simulink model "stewart_platform"  (R2013a)
settings: Solver=ode45  StartTime=0.0  StopTime=10.0  RelTol=1e-3
undefined symbols (not defined in the file): X, Y, Z
libraries: sm_lib x1374, nesl_utility x1
(part 22 of 30)

== system stewart_platform/ActuatorAssm4_2/DrivenAssm_1_RIGID/Recessed_Pan_Head_Screw_M2x8_48_Z_3_RIGID ==
  ReferenceFrame : sm_lib/Frames and  Transforms/Reference  Frame  BlockFunction=simmechanics.library.frames_transforms.reference_frame
  Solid : sm_lib/Body Elements/Solid  InertiaType=Custom  Mass=0.00030420099999999998  MassUnits=kg  CenterOfMass=[0.23057999999999998 -4.2158300000000003e-10 -1.6472500000000001e-11]  CenterOfMassUnits=cm  MomentsOfInertia=[3.0540999999999997e-06 2.6916499999999999e-05 2.6916499999999999e-05]  MomentsOfInertiaUnits=kg*cm^2  ProductsOfInertia=[0 0 0]  ProductsOfInertiaUnits=kg*cm^2  DensityBased=on  Density=1000  DensityUnits=kg/(m^3)  GraphicType=FromGeometry  MarkerShape=Sphere  MarkerSize=10  MarkerSizeUnits=m  GraphicVisPropType=SimpleVisualProperties  GraphicDiffuseColor=[0.722824 0.722824 0.722824]  GraphicSpecularColor=[0.5 0.5 0.5 1.0]  GraphicAmbientColor=[0.15 0.15 0.15 1.0]  GraphicEmissiveColor=[0.0 0.0 0.0 1.0]  GraphicShininess=75  GraphicOpacity=1  GeometryShape=FromFile  RectangleSize=[1 1]  RectangleSizeUnits=m  BrickDimensions=[1 1 1]  BrickDimensionUnits=m  CylinderRadius=1  CylinderRadiusUnits=m  CylinderLength=1  CylinderLengthUnits=m  SphereRadius=1  SphereRadiusUnits=m  EllipsoidRadii=[1 1 1]  EllipsoidRadiiUnits=m  ExtrusionCrossSection=[1 1; -1 1; -1 -1; 1 -1]  ExtrusionCrossSectionUnits=m  ExtrusionLength=1  ExtrusionLengthUnits=m  PolygonNumSides=3  PolygonOuterRadius=1  PolygonOuterRadiusUnits=m  ExtGeomFileName=Recessed_Pan_Head_Screw_M2x8_48_Z_Default_sldprt.STL  ExtGeomFileUnits=cm  RevolutionCrossSection=[1 1; 1 -1; 2 -1; 2 1]  RevolutionCrossSectionUnits=m  RevolutionExtent=Full  RevolutionAngle=180  RevolutionAngleUnits=deg  BlockFunction=simmechanics.library.body_elements.solid
  F : PMIOPort  Port=1  Side=Left
  connections:
  Solid/RConn1 -- ReferenceFrame/RConn1 -- F/RConn1

== system stewart_platform/ActuatorAssm4_2/DrivenAssm_1_RIGID/Recessed_Pan_Head_Screw_M2x8_48_Z_4_RIGID ==
  ReferenceFrame : sm_lib/Frames and  Transforms/Reference  Frame  BlockFunction=simmechanics.library.frames_transforms.reference_frame
  Solid : sm_lib/Body Elements/Solid  InertiaType=Custom  Mass=0.00030420099999999998  MassUnits=kg  CenterOfMass=[0.23057999999999998 -4.2158300000000003e-10 -1.6472500000000001e-11]  CenterOfMassUnits=cm  MomentsOfInertia=[3.0540999999999997e-06 2.6916499999999999e-05 2.6916499999999999e-05]  MomentsOfInertiaUnits=kg*cm^2  ProductsOfInertia=[0 0 0]  ProductsOfInertiaUnits=kg*cm^2  DensityBased=on  Density=1000  DensityUnits=kg/(m^3)  GraphicType=FromGeometry  MarkerShape=Sphere  MarkerSize=10  MarkerSizeUnits=m  GraphicVisPropType=SimpleVisualProperties  GraphicDiffuseColor=[0.722824 0.722824 0.722824]  GraphicSpecularColor=[0.5 0.5 0.5 1.0]  GraphicAmbientColor=[0.15 0.15 0.15 1.0]  GraphicEmissiveColor=[0.0 0.0 0.0 1.0]  GraphicShininess=75  GraphicOpacity=1  GeometryShape=FromFile  RectangleSize=[1 1]  RectangleSizeUnits=m  BrickDimensions=[1 1 1]  BrickDimensionUnits=m  CylinderRadius=1  CylinderRadiusUnits=m  CylinderLength=1  CylinderLengthUnits=m  SphereRadius=1  SphereRadiusUnits=m  EllipsoidRadii=[1 1 1]  EllipsoidRadiiUnits=m  ExtrusionCrossSection=[1 1; -1 1; -1 -1; 1 -1]  ExtrusionCrossSectionUnits=m  ExtrusionLength=1  ExtrusionLengthUnits=m  PolygonNumSides=3  PolygonOuterRadius=1  PolygonOuterRadiusUnits=m  ExtGeomFileName=Recessed_Pan_Head_Screw_M2x8_48_Z_Default_sldprt.STL  ExtGeomFileUnits=cm  RevolutionCrossSection=[1 1; 1 -1; 2 -1; 2 1]  RevolutionCrossSectionUnits=m  RevolutionExtent=Full  RevolutionAngle=180  RevolutionAngleUnits=deg  BlockFunction=simmechanics.library.body_elements.solid
  F : PMIOPort  Port=1  Side=Left
  connections:
  Solid/RConn1 -- ReferenceFrame/RConn1 -- F/RConn1

== system stewart_platform/ActuatorAssm4_2/DrivenAssm_1_RIGID/Recessed_Pan_Head_Screw_M2x8_48_Z_5_RIGID ==
  ReferenceFrame : sm_lib/Frames and  Transforms/Reference  Frame  BlockFunction=simmechanics.library.frames_transforms.reference_frame
  Solid : sm_lib/Body Elements/Solid  InertiaType=Custom  Mass=0.00030420099999999998  MassUnits=kg  CenterOfMass=[0.23057999999999998 -4.2158300000000003e-10 -1.6472500000000001e-11]  CenterOfMassUnits=cm  MomentsOfInertia=[3.0540999999999997e-06 2.6916499999999999e-05 2.6916499999999999e-05]  MomentsOfInertiaUnits=kg*cm^2  ProductsOfInertia=[0 0 0]  ProductsOfInertiaUnits=kg*cm^2  DensityBased=on  Density=1000  DensityUnits=kg/(m^3)  GraphicType=FromGeometry  MarkerShape=Sphere  MarkerSize=10  MarkerSizeUnits=m  GraphicVisPropType=SimpleVisualProperties  GraphicDiffuseColor=[0.722824 0.722824 0.722824]  GraphicSpecularColor=[0.5 0.5 0.5 1.0]  GraphicAmbientColor=[0.15 0.15 0.15 1.0]  GraphicEmissiveColor=[0.0 0.0 0.0 1.0]  GraphicShininess=75  GraphicOpacity=1  GeometryShape=FromFile  RectangleSize=[1 1]  RectangleSizeUnits=m  BrickDimensions=[1 1 1]  BrickDimensionUnits=m  CylinderRadius=1  CylinderRadiusUnits=m  CylinderLength=1  CylinderLengthUnits=m  SphereRadius=1  SphereRadiusUnits=m  EllipsoidRadii=[1 1 1]  EllipsoidRadiiUnits=m  ExtrusionCrossSection=[1 1; -1 1; -1 -1; 1 -1]  ExtrusionCrossSectionUnits=m  ExtrusionLength=1  ExtrusionLengthUnits=m  PolygonNumSides=3  PolygonOuterRadius=1  PolygonOuterRadiusUnits=m  ExtGeomFileName=Recessed_Pan_Head_Screw_M2x8_48_Z_Default_sldprt.STL  ExtGeomFileUnits=cm  RevolutionCrossSection=[1 1; 1 -1; 2 -1; 2 1]  RevolutionCrossSectionUnits=m  RevolutionExtent=Full  RevolutionAngle=180  RevolutionAngleUnits=deg  BlockFunction=simmechanics.library.body_elements.solid
  F : PMIOPort  Port=1  Side=Left
  connections:
  Solid/RConn1 -- ReferenceFrame/RConn1 -- F/RConn1

== system stewart_platform/ActuatorAssm4_2/DrivenAssm_1_RIGID/Recessed_Pan_Head_Screw_M2x8_48_Z_6_RIGID ==
  ReferenceFrame : sm_lib/Frames and  Transforms/Reference  Frame  BlockFunction=simmechanics.library.frames_transforms.reference_frame
  Solid : sm_lib/Body Elements/Solid  InertiaType=Custom  Mass=0.00030420099999999998  MassUnits=kg  CenterOfMass=[0.23057999999999998 -4.2158300000000003e-10 -1.6472500000000001e-11]  CenterOfMassUnits=cm  MomentsOfInertia=[3.0540999999999997e-06 2.6916499999999999e-05 2.6916499999999999e-05]  MomentsOfInertiaUnits=kg*cm^2  ProductsOfInertia=[0 0 0]  ProductsOfInertiaUnits=kg*cm^2  DensityBased=on  Density=1000  DensityUnits=kg/(m^3)  GraphicType=FromGeometry  MarkerShape=Sphere  MarkerSize=10  MarkerSizeUnits=m  GraphicVisPropType=SimpleVisualProperties  GraphicDiffuseColor=[0.722824 0.722824 0.722824]  GraphicSpecularColor=[0.5 0.5 0.5 1.0]  GraphicAmbientColor=[0.15 0.15 0.15 1.0]  GraphicEmissiveColor=[0.0 0.0 0.0 1.0]  GraphicShininess=75  GraphicOpacity=1  GeometryShape=FromFile  RectangleSize=[1 1]  RectangleSizeUnits=m  BrickDimensions=[1 1 1]  BrickDimensionUnits=m  CylinderRadius=1  CylinderRadiusUnits=m  CylinderLength=1  CylinderLengthUnits=m  SphereRadius=1  SphereRadiusUnits=m  EllipsoidRadii=[1 1 1]  EllipsoidRadiiUnits=m  ExtrusionCrossSection=[1 1; -1 1; -1 -1; 1 -1]  ExtrusionCrossSectionUnits=m  ExtrusionLength=1  ExtrusionLengthUnits=m  PolygonNumSides=3  PolygonOuterRadius=1  PolygonOuterRadiusUnits=m  ExtGeomFileName=Recessed_Pan_Head_Screw_M2x8_48_Z_Default_sldprt.STL  ExtGeomFileUnits=cm  RevolutionCrossSection=[1 1; 1 -1; 2 -1; 2 1]  RevolutionCrossSectionUnits=m  RevolutionExtent=Full  RevolutionAngle=180  RevolutionAngleUnits=deg  BlockFunction=simmechanics.library.body_elements.solid
  F : PMIOPort  Port=1  Side=Left
  connections:
  Solid/RConn1 -- ReferenceFrame/RConn1 -- F/RConn1

== system stewart_platform/ActuatorAssm4_2/DrivenAssm_1_RIGID/Recessed_Pan_Head_Screw_M2x8_48_Z_7_RIGID ==
  ReferenceFrame : sm_lib/Frames and  Transforms/Reference  Frame  BlockFunction=simmechanics.library.frames_transforms.reference_frame
  Solid : sm_lib/Body Elements/Solid  InertiaType=Custom  Mass=0.00030420099999999998  MassUnits=kg  CenterOfMass=[0.23057999999999998 -4.2158300000000003e-10 -1.6472500000000001e-11]  CenterOfMassUnits=cm  MomentsOfInertia=[3.0540999999999997e-06 2.6916499999999999e-05 2.6916499999999999e-05]  MomentsOfInertiaUnits=kg*cm^2  ProductsOfInertia=[0 0 0]  ProductsOfInertiaUnits=kg*cm^2  DensityBased=on  Density=1000  DensityUnits=kg/(m^3)  GraphicType=FromGeometry  MarkerShape=Sphere  MarkerSize=10  MarkerSizeUnits=m  GraphicVisPropType=SimpleVisualProperties  GraphicDiffuseColor=[0.722824 0.722824 0.722824]  GraphicSpecularColor=[0.5 0.5 0.5 1.0]  GraphicAmbientColor=[0.15 0.15 0.15 1.0]  GraphicEmissiveColor=[0.0 0.0 0.0 1.0]  GraphicShininess=75  GraphicOpacity=1  GeometryShape=FromFile  RectangleSize=[1 1]  RectangleSizeUnits=m  BrickDimensions=[1 1 1]  BrickDimensionUnits=m  CylinderRadius=1  CylinderRadiusUnits=m  CylinderLength=1  CylinderLengthUnits=m  SphereRadius=1  SphereRadiusUnits=m  EllipsoidRadii=[1 1 1]  EllipsoidRadiiUnits=m  ExtrusionCrossSection=[1 1; -1 1; -1 -1; 1 -1]  ExtrusionCrossSectionUnits=m  ExtrusionLength=1  ExtrusionLengthUnits=m  PolygonNumSides=3  PolygonOuterRadius=1  PolygonOuterRadiusUnits=m  ExtGeomFileName=Recessed_Pan_Head_Screw_M2x8_48_Z_Default_sldprt.STL  ExtGeomFileUnits=cm  RevolutionCrossSection=[1 1; 1 -1; 2 -1; 2 1]  RevolutionCrossSectionUnits=m  RevolutionExtent=Full  RevolutionAngle=180  RevolutionAngleUnits=deg  BlockFunction=simmechanics.library.body_elements.solid
  F : PMIOPort  Port=1  Side=Left
  connections:
  Solid/RConn1 -- ReferenceFrame/RConn1 -- F/RConn1

== system stewart_platform/ActuatorAssm4_2/DrivenAssm_1_RIGID/Recessed_Pan_Head_Screw_M2x8_48_Z_8_RIGID ==
  ReferenceFrame : sm_lib/Frames and  Transforms/Reference  Frame  BlockFunction=simmechanics.library.frames_transforms.reference_frame
  Solid : sm_lib/Body Elements/Solid  InertiaType=Custom  Mass=0.00030420099999999998  MassUnits=kg  CenterOfMass=[0.23057999999999998 -4.2158300000000003e-10 -1.6472500000000001e-11]  CenterOfMassUnits=cm  MomentsOfInertia=[3.0540999999999997e-06 2.6916499999999999e-05 2.6916499999999999e-05]  MomentsOfInertiaUnits=kg*cm^2  ProductsOfInertia=[0 0 0]  ProductsOfInertiaUnits=kg*cm^2  DensityBased=on  Density=1000  DensityUnits=kg/(m^3)  GraphicType=FromGeometry  MarkerShape=Sphere  MarkerSize=10  MarkerSizeUnits=m  GraphicVisPropType=SimpleVisualProperties  GraphicDiffuseColor=[0.722824 0.722824 0.722824]  GraphicSpecularColor=[0.5 0.5 0.5 1.0]  GraphicAmbientColor=[0.15 0.15 0.15 1.0]  GraphicEmissiveColor=[0.0 0.0 0.0 1.0]  GraphicShininess=75  GraphicOpacity=1  GeometryShape=FromFile  RectangleSize=[1 1]  RectangleSizeUnits=m  BrickDimensions=[1 1 1]  BrickDimensionUnits=m  CylinderRadius=1  CylinderRadiusUnits=m  CylinderLength=1  CylinderLengthUnits=m  SphereRadius=1  SphereRadiusUnits=m  EllipsoidRadii=[1 1 1]  EllipsoidRadiiUnits=m  ExtrusionCrossSection=[1 1; -1 1; -1 -1; 1 -1]  ExtrusionCrossSectionUnits=m  ExtrusionLength=1  ExtrusionLengthUnits=m  PolygonNumSides=3  PolygonOuterRadius=1  PolygonOuterRadiusUnits=m  ExtGeomFileName=Recessed_Pan_Head_Screw_M2x8_48_Z_Default_sldprt.STL  ExtGeomFileUnits=cm  RevolutionCrossSection=[1 1; 1 -1; 2 -1; 2 1]  RevolutionCrossSectionUnits=m  RevolutionExtent=Full  RevolutionAngle=180  RevolutionAngleUnits=deg  BlockFunction=simmechanics.library.body_elements.solid
  F : PMIOPort  Port=1  Side=Left
  connections:
  Solid/RConn1 -- ReferenceFrame/RConn1 -- F/RConn1

== system stewart_platform/ActuatorAssm4_2/DrivenAssm_1_RIGID/Recessed_Pan_Head_Screw_M2x8_48_Z_9_RIGID ==
  ReferenceFrame : sm_lib/Frames and  Transforms/Reference  Frame  BlockFunction=simmechanics.library.frames_transforms.reference_frame
  Solid : sm_lib/Body Elements/Solid  InertiaType=Custom  Mass=0.00030420099999999998  MassUnits=kg  CenterOfMass=[0.23057999999999998 -4.2158300000000003e-10 -1.6472500000000001e-11]  CenterOfMassUnits=cm  MomentsOfInertia=[3.0540999999999997e-06 2.6916499999999999e-05 2.6916499999999999e-05]  MomentsOfInertiaUnits=kg*cm^2  ProductsOfInertia=[0 0 0]  ProductsOfInertiaUnits=kg*cm^2  DensityBased=on  Density=1000  DensityUnits=kg/(m^3)  GraphicType=FromGeometry  MarkerShape=Sphere  MarkerSize=10  MarkerSizeUnits=m  GraphicVisPropType=SimpleVisualProperties  GraphicDiffuseColor=[0.722824 0.722824 0.722824]  GraphicSpecularColor=[0.5 0.5 0.5 1.0]  GraphicAmbientColor=[0.15 0.15 0.15 1.0]  GraphicEmissiveColor=[0.0 0.0 0.0 1.0]  GraphicShininess=75  GraphicOpacity=1  GeometryShape=FromFile  RectangleSize=[1 1]  RectangleSizeUnits=m  BrickDimensions=[1 1 1]  BrickDimensionUnits=m  CylinderRadius=1  CylinderRadiusUnits=m  CylinderLength=1  CylinderLengthUnits=m  SphereRadius=1  SphereRadiusUnits=m  EllipsoidRadii=[1 1 1]  EllipsoidRadiiUnits=m  ExtrusionCrossSection=[1 1; -1 1; -1 -1; 1 -1]  ExtrusionCrossSectionUnits=m  ExtrusionLength=1  ExtrusionLengthUnits=m  PolygonNumSides=3  PolygonOuterRadius=1  PolygonOuterRadiusUnits=m  ExtGeomFileName=Recessed_Pan_Head_Screw_M2x8_48_Z_Default_sldprt.STL  ExtGeomFileUnits=cm  RevolutionCrossSection=[1 1; 1 -1; 2 -1; 2 1]  RevolutionCrossSectionUnits=m  RevolutionExtent=Full  RevolutionAngle=180  RevolutionAngleUnits=deg  BlockFunction=simmechanics.library.body_elements.solid
  F : PMIOPort  Port=1  Side=Left
  connections:
  Solid/RConn1 -- ReferenceFrame/RConn1 -- F/RConn1

== system stewart_platform/ActuatorAssm4_2/DrivenAssm_1_RIGID/SV2075_1_RIGID ==
  ReferenceFrame : sm_lib/Frames and  Transforms/Reference  Frame  BlockFunction=simmechanics.library.frames_transforms.reference_frame
  Solid : sm_lib/Body Elements/Solid  InertiaType=Custom  Mass=0.0058459100000000002  MassUnits=kg  CenterOfMass=[-0.32989499999999999 0.0096923500000000006 3.75]  CenterOfMassUnits=cm  MomentsOfInertia=[0.027698799999999999 0.027673900000000001 0.00032823000000000005]  MomentsOfInertiaUnits=kg*cm^2  ProductsOfInertia=[0 0 -1.1416499999999999e-06]  ProductsOfInertiaUnits=kg*cm^2  DensityBased=on  Density=1000  DensityUnits=kg/(m^3)  GraphicType=FromGeometry  MarkerShape=Sphere  MarkerSize=10  MarkerSizeUnits=m  GraphicVisPropType=SimpleVisualProperties  GraphicDiffuseColor=[0.98 0.98 0.98]  GraphicSpecularColor=[0.5 0.5 0.5 1.0]  GraphicAmbientColor=[0.15 0.15 0.15 1.0]  GraphicEmissiveColor=[0.0 0.0 0.0 1.0]  GraphicShininess=75  GraphicOpacity=1  GeometryShape=FromFile  RectangleSize=[1 1]  RectangleSizeUnits=m  BrickDimensions=[1 1 1]  BrickDimensionUnits=m  CylinderRadius=1  CylinderRadiusUnits=m  CylinderLength=1  CylinderLengthUnits=m  SphereRadius=1  SphereRadiusUnits=m  EllipsoidRadii=[1 1 1]  EllipsoidRadiiUnits=m  ExtrusionCrossSection=[1 1; -1 1; -1 -1; 1 -1]  ExtrusionCrossSectionUnits=m  ExtrusionLength=1  ExtrusionLengthUnits=m  PolygonNumSides=3  PolygonOuterRadius=1  PolygonOuterRadiusUnits=m  ExtGeomFileName=SV2075_Default_sldprt.STL  ExtGeomFileUnits=cm  RevolutionCrossSection=[1 1; 1 -1; 2 -1; 2 1]  RevolutionCrossSectionUnits=m  RevolutionExtent=Full  RevolutionAngle=180  RevolutionAngleUnits=deg  BlockFunction=simmechanics.library.body_elements.solid
  F : PMIOPort  Port=1  Side=Left
  connections:
  Solid/RConn1 -- ReferenceFrame/RConn1 -- F/RConn1

== system stewart_platform/ActuatorAssm4_2/DrivenAssm_1_RIGID/SV2075_2_RIGID ==
  ReferenceFrame : sm_lib/Frames and  Transforms/Reference  Frame  BlockFunction=simmechanics.library.frames_transforms.reference_frame
  Solid : sm_lib/Body Elements/Solid  InertiaType=Custom  Mass=0.0058459100000000002  MassUnits=kg  CenterOfMass=[-0.32989499999999999 0.0096923500000000006 3.75]  CenterOfMassUnits=cm  MomentsOfInertia=[0.027698799999999999 0.027673900000000001 0.00032823000000000005]  MomentsOfInertiaUnits=kg*cm^2  ProductsOfInertia=[0 0 -1.1416499999999999e-06]  ProductsOfInertiaUnits=kg*cm^2  DensityBased=on  Density=1000  DensityUnits=kg/(m^3)  GraphicType=FromGeometry  MarkerShape=Sphere  MarkerSize=10  MarkerSizeUnits=m  GraphicVisPropType=SimpleVisualProperties  GraphicDiffuseColor=[0.98 0.98 0.98]  GraphicSpecularColor=[0.5 0.5 0.5 1.0]  GraphicAmbientColor=[0.15 0.15 0.15 1.0]  GraphicEmissiveColor=[0.0 0.0 0.0 1.0]  GraphicShininess=75  GraphicOpacity=1  GeometryShape=FromFile  RectangleSize=[1 1]  RectangleSizeUnits=m  BrickDimensions=[1 1 1]  BrickDimensionUnits=m  CylinderRadius=1  CylinderRadiusUnits=m  CylinderLength=1  CylinderLengthUnits=m  SphereRadius=1  SphereRadiusUnits=m  EllipsoidRadii=[1 1 1]  EllipsoidRadiiUnits=m  ExtrusionCrossSection=[1 1; -1 1; -1 -1; 1 -1]  ExtrusionCrossSectionUnits=m  ExtrusionLength=1  ExtrusionLengthUnits=m  PolygonNumSides=3  PolygonOuterRadius=1  PolygonOuterRadiusUnits=m  ExtGeomFileName=SV2075_Default_sldprt.STL  ExtGeomFileUnits=cm  RevolutionCrossSection=[1 1; 1 -1; 2 -1; 2 1]  RevolutionCrossSectionUnits=m  RevolutionExtent=Full  RevolutionAngle=180  RevolutionAngleUnits=deg  BlockFunction=simmechanics.library.body_elements.solid
  F : PMIOPort  Port=1  Side=Left
  connections:
  Solid/RConn1 -- ReferenceFrame/RConn1 -- F/RConn1

== system stewart_platform/ActuatorAssm4_2/DrivenAssm_1_RIGID/Yoke_1_RIGID ==
  ReferenceFrame : sm_lib/Frames and  Transforms/Reference  Frame  BlockFunction=simmechanics.library.frames_transforms.reference_frame
  Solid : sm_lib/Body Elements/Solid  InertiaType=Custom  Mass=0.0085668099999999994  MassUnits=kg  CenterOfMass=[3.3036099999999999e-09 4.5392100000000001e-09 0.0138091]  CenterOfMassUnits=m  MomentsOfInertia=[3.6198600000000002e-07 3.7260700000000002e-07 1.1777300000000001e-07]  MomentsOfInertiaUnits=kg*m^2  ProductsOfInertia=[-1.58919e-13 -3.9281799999999999e-13 1.96468e-13]  ProductsOfInertiaUnits=kg*m^2  DensityBased=on  Density=1000  DensityUnits=kg/(m^3)  GraphicType=FromGeometry  MarkerShape=Sphere  MarkerSize=10  MarkerSizeUnits=m  GraphicVisPropType=SimpleVisualProperties  GraphicDiffuseColor=[0.594824 0.594824 0.594824]  GraphicSpecularColor=[0.5 0.5 0.5 1.0]  GraphicAmbientColor=[0.15 0.15 0.15 1.0]  GraphicEmissiveColor=[0.0 0.0 0.0 1.0]  GraphicShininess=75  GraphicOpacity=1  GeometryShape=FromFile  RectangleSize=[1 1]  RectangleSizeUnits=m  BrickDimensions=[1 1 1]  BrickDimensionUnits=m  CylinderRadius=1  CylinderRadiusUnits=m  CylinderLength=1  CylinderLengthUnits=m  SphereRadius=1  SphereRadiusUnits=m  EllipsoidRadii=[1 1 1]  EllipsoidRadiiUnits=m  ExtrusionCrossSection=[1 1; -1 1; -1 -1; 1 -1]  ExtrusionCrossSectionUnits=m  ExtrusionLength=1  ExtrusionLengthUnits=m  PolygonNumSides=3  PolygonOuterRadius=1  PolygonOuterRadiusUnits=m  ExtGeomFileName=Yoke_Default_sldprt.STL  ExtGeomFileUnits=m  RevolutionCrossSection=[1 1; 1 -1; 2 -1; 2 1]  RevolutionCrossSectionUnits=m  RevolutionExtent=Full  RevolutionAngle=180  RevolutionAngleUnits=deg  BlockFunction=simmechanics.library.body_elements.solid
  F : PMIOPort  Port=1  Side=Left
  connections:
  Solid/RConn1 -- ReferenceFrame/RConn1 -- F/RConn1

== system stewart_platform/ActuatorAssm4_2/DrivenAssm_1_RIGID/pin2_1_RIGID ==
  ReferenceFrame : sm_lib/Frames and  Transforms/Reference  Frame  BlockFunction=simmechanics.library.frames_transforms.reference_frame
  Solid : sm_lib/Body Elements/Solid  InertiaType=Custom  Mass=0.00306405  MassUnits=kg  CenterOfMass=[0.62878100000000003 1.2281900000000002e-05 9.2878900000000002e-08]  CenterOfMassUnits=cm  MomentsOfInertia=[0.00015143299999999997 0.00047164 0.000471626]  MomentsOfInertiaUnits=kg*cm^2  ProductsOfInertia=[9.4727800000000005e-10 -1.42807e-10 -1.8883699999999999e-08]  ProductsOfInertiaUnits=kg*cm^2  DensityBased=on  Density=1000  DensityUnits=kg/(m^3)  GraphicType=FromGeometry  MarkerShape=Sphere  MarkerSize=10  MarkerSizeUnits=m  GraphicVisPropType=SimpleVisualProperties  GraphicDiffuseColor=[0.722824 0.722824 0.722824]  GraphicSpecularColor=[0.5 0.5 0.5 1.0]  GraphicAmbientColor=[0.15 0.15 0.15 1.0]  GraphicEmissiveColor=[0.0 0.0 0.0 1.0]  GraphicShininess=75  GraphicOpacity=1  GeometryShape=FromFile  RectangleSize=[1 1]  RectangleSizeUnits=m  BrickDimensions=[1 1 1]  BrickDimensionUnits=m  CylinderRadius=1  CylinderRadiusUnits=m  CylinderLength=1  CylinderLengthUnits=m  SphereRadius=1  SphereRadiusUnits=m  EllipsoidRadii=[1 1 1]  EllipsoidRadiiUnits=m  ExtrusionCrossSection=[1 1; -1 1; -1 -1; 1 -1]  ExtrusionCrossSectionUnits=m  ExtrusionLength=1  ExtrusionLengthUnits=m  PolygonNumSides=3  PolygonOuterRadius=1  PolygonOuterRadiusUnits=m  ExtGeomFileName=pin2_Default_sldprt.STL  ExtGeomFileUnits=cm  RevolutionCrossSection=[1 1; 1 -1; 2 -1; 2 1]  RevolutionCrossSectionUnits=m  RevolutionExtent=Full  RevolutionAngle=180  RevolutionAngleUnits=deg  BlockFunction=simmechanics.library.body_elements.solid
  F : PMIOPort  Port=1  Side=Left
  connections:
  Solid/RConn1 -- ReferenceFrame/RConn1 -- F/RConn1

== system stewart_platform/ActuatorAssm5_2/CarrierAssm_1_RIGID/Carrier_Block_1_RIGID ==
  ReferenceFrame : sm_lib/Frames and  Transforms/Reference  Frame  BlockFunction=simmechanics.library.frames_transforms.reference_frame
  Solid : sm_lib/Body Elements/Solid  InertiaType=Custom  Mass=0.29755500000000001  MassUnits=kg  CenterOfMass=[0.052371599999999997 -0.00023156000000000001 0.0090326099999999999]  CenterOfMassUnits=m  MomentsOfInertia=[0.000116325 0.000380615 0.00046776100000000002]  MomentsOfInertiaUnits=kg*m^2  ProductsOfInertia=[7.7054000000000002e-07 8.2627199999999994e-06 5.2656100000000005e-07]  ProductsOfInertiaUnits=kg*m^2  DensityBased=on  Density=1000  DensityUnits=kg/(m^3)  GraphicType=FromGeometry  MarkerShape=Sphere  MarkerSize=10  MarkerSizeUnits=m  GraphicVisPropType=SimpleVisualProperties  GraphicDiffuseColor=[0.215686 0.607843 1]  GraphicSpecularColor=[0.5 0.5 0.5 1.0]  GraphicAmbientColor=[0.15 0.15 0.15 1.0]  GraphicEmissiveColor=[0.0 0.0 0.0 1.0]  GraphicShininess=75  GraphicOpacity=1  GeometryShape=FromFile  RectangleSize=[1 1]  RectangleSizeUnits=m  BrickDimensions=[1 1 1]  BrickDimensionUnits=m  CylinderRadius=1  CylinderRadiusUnits=m  CylinderLength=1  CylinderLengthUnits=m  SphereRadius=1  SphereRadiusUnits=m  EllipsoidRadii=[1 1 1]  EllipsoidRadiiUnits=m  ExtrusionCrossSection=[1 1; -1 1; -1 -1; 1 -1]  ExtrusionCrossSectionUnits=m  ExtrusionLength=1  ExtrusionLengthUnits=m  PolygonNumSides=3  PolygonOuterRadius=1  PolygonOuterRadiusUnits=m  ExtGeomFileName=Carrier_Block_Default_sldprt.STL  ExtGeomFileUnits=m  RevolutionCrossSection=[1 1; 1 -1; 2 -1; 2 1]  RevolutionCrossSectionUnits=m  RevolutionExtent=Full  RevolutionAngle=180  RevolutionAngleUnits=deg  BlockFunction=simmechanics.library.body_elements.solid
  F : PMIOPort  Port=1  Side=Left
  connections:
  Solid/RConn1 -- ReferenceFrame/RConn1 -- F/RConn1

== system stewart_platform/ActuatorAssm5_2/CarrierAssm_1_RIGID/Cylinder_Head_Cap_Screw_M3x8_1_RIGID ==
  ReferenceFrame : sm_lib/Frames and  Transforms/Reference  Frame  BlockFunction=simmechanics.library.frames_transforms.reference_frame
  Solid : sm_lib/Body Elements/Solid  InertiaType=Custom  Mass=0.000756816  MassUnits=kg  CenterOfMass=[0.18814900000000001 4.2404900000000005e-05 3.03142e-07]  CenterOfMassUnits=cm  MomentsOfInertia=[1.84419e-05 7.8615999999999994e-05 7.8603699999999987e-05]  MomentsOfInertiaUnits=kg*cm^2  ProductsOfInertia=[8.2955699999999995e-10 -6.6108000000000001e-11 -9.2474899999999991e-09]  ProductsOfInertiaUnits=kg*cm^2  DensityBased=on  Density=1000  DensityUnits=kg/(m^3)  GraphicType=FromGeometry  MarkerShape=Sphere  MarkerSize=10  MarkerSizeUnits=m  GraphicVisPropType=SimpleVisualProperties  GraphicDiffuseColor=[0.722824 0.722824 0.722824]  GraphicSpecularColor=[0.5 0.5 0.5 1.0]  GraphicAmbientColor=[0.15 0.15 0.15 1.0]  GraphicEmissiveColor=[0.0 0.0 0.0 1.0]  GraphicShininess=75  GraphicOpacity=1  GeometryShape=FromFile  RectangleSize=[1 1]  RectangleSizeUnits=m  BrickDimensions=[1 1 1]  BrickDimensionUnits=m  CylinderRadius=1  CylinderRadiusUnits=m  CylinderLength=1  CylinderLengthUnits=m  SphereRadius=1  SphereRadiusUnits=m  EllipsoidRadii=[1 1 1]  EllipsoidRadiiUnits=m  ExtrusionCrossSection=[1 1; -1 1; -1 -1; 1 -1]  ExtrusionCrossSectionUnits=m  ExtrusionLength=1  ExtrusionLengthUnits=m  PolygonNumSides=3  PolygonOuterRadius=1  PolygonOuterRadiusUnits=m  ExtGeomFileName=Cylinder_Head_Cap_Screw_M3x8_Default_sldprt.STL  ExtGeomFileUnits=cm  RevolutionCrossSection=[1 1; 1 -1; 2 -1; 2 1]  RevolutionCrossSectionUnits=m  RevolutionExtent=Full  RevolutionAngle=180  RevolutionAngleUnits=deg  BlockFunction=simmechanics.library.body_elements.solid
  F : PMIOPort  Port=1  Side=Left
  connections:
  Solid/RConn1 -- ReferenceFrame/RConn1 -- F/RConn1

== system stewart_platform/ActuatorAssm5_2/CarrierAssm_1_RIGID/Cylinder_Head_Cap_Screw_M3x8_2_RIGID ==
  ReferenceFrame : sm_lib/Frames and  Transforms/Reference  Frame  BlockFunction=simmechanics.library.frames_transforms.reference_frame
  Solid : sm_lib/Body Elements/Solid  InertiaType=Custom  Mass=0.000756816  MassUnits=kg  CenterOfMass=[0.18814900000000001 4.2404900000000005e-05 3.03142e-07]  CenterOfMassUnits=cm  MomentsOfInertia=[1.84419e-05 7.8615999999999994e-05 7.8603699999999987e-05]  MomentsOfInertiaUnits=kg*cm^2  ProductsOfInertia=[8.2955699999999995e-10 -6.6108000000000001e-11 -9.2474899999999991e-09]  ProductsOfInertiaUnits=kg*cm^2  DensityBased=on  Density=1000  DensityUnits=kg/(m^3)  GraphicType=FromGeometry  MarkerShape=Sphere  MarkerSize=10  MarkerSizeUnits=m  GraphicVisPropType=SimpleVisualProperties  GraphicDiffuseColor=[0.722824 0.722824 0.722824]  GraphicSpecularColor=[0.5 0.5 0.5 1.0]  GraphicAmbientColor=[0.15 0.15 0.15 1.0]  GraphicEmissiveColor=[0.0 0.0 0.0 1.0]  GraphicShininess=75  GraphicOpacity=1  GeometryShape=FromFile  RectangleSize=[1 1]  RectangleSizeUnits=m  BrickDimensions=[1 1 1]  BrickDimensionUnits=m  CylinderRadius=1  CylinderRadiusUnits=m  CylinderLength=1  CylinderLengthUnits=m  SphereRadius=1  SphereRadiusUnits=m  EllipsoidRadii=[1 1 1]  EllipsoidRadiiUnits=m  ExtrusionCrossSection=[1 1; -1 1; -1 -1; 1 -1]  ExtrusionCrossSectionUnits=m  ExtrusionLength=1  ExtrusionLengthUnits=m  PolygonNumSides=3  PolygonOuterRadius=1  PolygonOuterRadiusUnits=m  ExtGeomFileName=Cylinder_Head_Cap_Screw_M3x8_Default_sldprt.STL  ExtGeomFileUnits=cm  RevolutionCrossSection=[1 1; 1 -1; 2 -1; 2 1]  RevolutionCrossSectionUnits=m  RevolutionExtent=Full  RevolutionAngle=180  RevolutionAngleUnits=deg  BlockFunction=simmechanics.library.body_elements.solid
  F : PMIOPort  Port=1  Side=Left
  connections:
  Solid/RConn1 -- ReferenceFrame/RConn1 -- F/RConn1

== system stewart_platform/ActuatorAssm5_2/CarrierAssm_1_RIGID/HR_1_Motor_1_RIGID ==
  ReferenceFrame : sm_lib/Frames and  Transforms/Reference  Frame  BlockFunction=simmechanics.library.frames_transforms.reference_frame
  Solid : sm_lib/Body Elements/Solid  InertiaType=Custom  Mass=0.016323299999999999  MassUnits=kg  CenterOfMass=[1.14618 1.9088000000000001 0.39999800000000002]  CenterOfMassUnits=cm  MomentsOfInertia=[0.022976199999999999 0.016967199999999998 0.038272499999999994]  MomentsOfInertiaUnits=kg*cm^2  ProductsOfInertia=[6.3449800000000005e-08 1.4415399999999998e-07 0.0031628799999999999]  ProductsOfInertiaUnits=kg*cm^2  DensityBased=on  Density=1000  DensityUnits=kg/(m^3)  GraphicType=FromGeometry  MarkerShape=Sphere  MarkerSize=10  MarkerSizeUnits=m  GraphicVisPropType=SimpleVisualProperties  GraphicDiffuseColor=[0.96 0.696471 0.568471]  GraphicSpecularColor=[0.5 0.5 0.5 1.0]  GraphicAmbientColor=[0.15 0.15 0.15 1.0]  GraphicEmissiveColor=[0.0 0.0 0.0 1.0]  GraphicShininess=75  GraphicOpacity=1  GeometryShape=FromFile  RectangleSize=[1 1]  RectangleSizeUnits=m  BrickDimensions=[1 1 1]  BrickDimensionUnits=m  CylinderRadius=1  CylinderRadiusUnits=m  CylinderLength=1  CylinderLengthUnits=m  SphereRadius=1  SphereRadiusUnits=m  EllipsoidRadii=[1 1 1]  EllipsoidRadiiUnits=m  ExtrusionCrossSection=[1 1; -1 1; -1 -1; 1 -1]  ExtrusionCrossSectionUnits=m  ExtrusionLength=1  ExtrusionLengthUnits=m  PolygonNumSides=3  PolygonOuterRadius=1  PolygonOuterRadiusUnits=m  ExtGeomFileName=HR_1_Motor_Default_sldprt.STL  ExtGeomFileUnits=cm  RevolutionCrossSection=[1 1; 1 -1; 2 -1; 2 1]  RevolutionCrossSectionUnits=m  RevolutionExtent=Full  RevolutionAngle=180  RevolutionAngleUnits=deg  BlockFunction=simmechanics.library.body_elements.solid
  F : PMIOPort  Port=1  Side=Left
  connections:
  Solid/RConn1 -- ReferenceFrame/RConn1 -- F/RConn1

== system stewart_platform/ActuatorAssm5_2/CarrierAssm_1_RIGID/HR_1_Motor_2_RIGID ==
  ReferenceFrame : sm_lib/Frames and  Transforms/Reference  Frame  BlockFunction=simmechanics.library.frames_transforms.reference_frame
  Solid : sm_lib/Body Elements/Solid  InertiaType=Custom  Mass=0.016323299999999999  MassUnits=kg  CenterOfMass=[1.14618 1.9088000000000001 0.39999800000000002]  CenterOfMassUnits=cm  MomentsOfInertia=[0.022976199999999999 0.016967199999999998 0.038272499999999994]  MomentsOfInertiaUnits=kg*cm^2  ProductsOfInertia=[6.3449800000000005e-08 1.4415399999999998e-07 0.0031628799999999999]  ProductsOfInertiaUnits=kg*cm^2  DensityBased=on  Density=1000  DensityUnits=kg/(m^3)  GraphicType=FromGeometry  MarkerShape=Sphere  MarkerSize=10  MarkerSizeUnits=m  GraphicVisPropType=SimpleVisualProperties  GraphicDiffuseColor=[0.96 0.696471 0.568471]  GraphicSpecularColor=[0.5 0.5 0.5 1.0]  GraphicAmbientColor=[0.15 0.15 0.15 1.0]  GraphicEmissiveColor=[0.0 0.0 0.0 1.0]  GraphicShininess=75  GraphicOpacity=1  GeometryShape=FromFile  RectangleSize=[1 1]  RectangleSizeUnits=m  BrickDimensions=[1 1 1]  BrickDimensionUnits=m  CylinderRadius=1  CylinderRadiusUnits=m  CylinderLength=1  CylinderLengthUnits=m  SphereRadius=1  SphereRadiusUnits=m  EllipsoidRadii=[1 1 1]  EllipsoidRadiiUnits=m  ExtrusionCrossSection=[1 1; -1 1; -1 -1; 1 -1]  ExtrusionCrossSectionUnits=m  ExtrusionLength=1  ExtrusionLengthUnits=m  PolygonNumSides=3  PolygonOuterRadius=1  PolygonOuterRadiusUnits=m  ExtGeomFileName=HR_1_Motor_Default_sldprt.STL  ExtGeomFileUnits=cm  RevolutionCrossSection=[1 1; 1 -1; 2 -1; 2 1]  RevolutionCrossSectionUnits=m  RevolutionExtent=Full  RevolutionAngle=180  RevolutionAngleUnits=deg  BlockFunction=simmechanics.library.body_elements.solid
  F : PMIOPort  Port=1  Side=Left
  connections:
  Solid/RConn1 -- ReferenceFrame/RConn1 -- F/RConn1

== system stewart_platform/ActuatorAssm5_2/CarrierAssm_1_RIGID/Hexagon_Socket_Button_Head_Screw_M3x6_1_RIGID ==
  ReferenceFrame : sm_lib/Frames and  Transforms/Reference  Frame  BlockFunction=simmechanics.library.frames_transforms.reference_frame
  Solid : sm_lib/Body Elements/Solid  InertiaType=Custom  Mass=0.00056348200000000002  MassUnits=kg  CenterOfMass=[0.143563 8.1476600000000005e-06 5.87883e-08]  CenterOfMassUnits=cm  MomentsOfInertia=[1.3098999999999999e-05 3.5078399999999999e-05 3.5077400000000004e-05]  MomentsOfInertiaUnits=kg*cm^2  ProductsOfInertia=[6.7519100000000001e-11 -7.6873799999999995e-12 -1.06542e-09]  ProductsOfInertiaUnits=kg*cm^2  DensityBased=on  Density=1000  DensityUnits=kg/(m^3)  GraphicType=FromGeometry  MarkerShape=Sphere  MarkerSize=10  MarkerSizeUnits=m  GraphicVisPropType=SimpleVisualProperties  GraphicDiffuseColor=[0.722824 0.722824 0.722824]  GraphicSpecularColor=[0.5 0.5 0.5 1.0]  GraphicAmbientColor=[0.15 0.15 0.15 1.0]  GraphicEmissiveColor=[0.0 0.0 0.0 1.0]  GraphicShininess=75  GraphicOpacity=1  GeometryShape=FromFile  RectangleSize=[1 1]  RectangleSizeUnits=m  BrickDimensions=[1 1 1]  BrickDimensionUnits=m  CylinderRadius=1  CylinderRadiusUnits=m  CylinderLength=1  CylinderLengthUnits=m  SphereRadius=1  SphereRadiusUnits=m  EllipsoidRadii=[1 1 1]  EllipsoidRadiiUnits=m  ExtrusionCrossSection=[1 1; -1 1; -1 -1; 1 -1]  ExtrusionCrossSectionUnits=m  ExtrusionLength=1  ExtrusionLengthUnits=m  PolygonNumSides=3  PolygonOuterRadius=1  PolygonOuterRadiusUnits=m  ExtGeomFileName=Hexagon_Socket_Button_Head_Screw_M3x6_Default_sldprt.STL  ExtGeomFileUnits=cm  RevolutionCrossSection=[1 1; 1 -1; 2 -1; 2 1]  RevolutionCrossSectionUnits=m  RevolutionExtent=Full  RevolutionAngle=180  RevolutionAngleUnits=deg  BlockFunction=simmechanics.library.body_elements.solid
  F : PMIOPort  Port=1  Side=Left
  connections:
  Solid/RConn1 -- ReferenceFrame/RConn1 -- F/RConn1

== system stewart_platform/ActuatorAssm5_2/CarrierAssm_1_RIGID/Hexagon_Socket_Button_Head_Screw_M3x6_2_RIGID ==
  ReferenceFrame : sm_lib/Frames and  Transforms/Reference  Frame  BlockFunction=simmechanics.library.frames_transforms.reference_frame
  Solid : sm_lib/Body Elements/Solid  InertiaType=Custom  Mass=0.00056348200000000002  MassUnits=kg  CenterOfMass=[0.143563 8.1476600000000005e-06 5.87883e-08]  CenterOfMassUnits=cm  MomentsOfInertia=[1.3098999999999999e-05 3.5078399999999999e-05 3.5077400000000004e-05]  MomentsOfInertiaUnits=kg*cm^2  ProductsOfInertia=[6.7519100000000001e-11 -7.6873799999999995e-12 -1.06542e-09]  ProductsOfInertiaUnits=kg*cm^2  DensityBased=on  Density=1000  DensityUnits=kg/(m^3)  GraphicType=FromGeometry  MarkerShape=Sphere  MarkerSize=10  MarkerSizeUnits=m  GraphicVisPropType=SimpleVisualProperties  GraphicDiffuseColor=[0.722824 0.722824 0.722824]  GraphicSpecularColor=[0.5 0.5 0.5 1.0]  GraphicAmbientColor=[0.15 0.15 0.15 1.0]  GraphicEmissiveColor=[0.0 0.0 0.0 1.0]  GraphicShininess=75  GraphicOpacity=1  GeometryShape=FromFile  RectangleSize=[1 1]  RectangleSizeUnits=m  BrickDimensions=[1 1 1]  BrickDimensionUnits=m  CylinderRadius=1  CylinderRadiusUnits=m  CylinderLength=1  CylinderLengthUnits=m  SphereRadius=1  SphereRadiusUnits=m  EllipsoidRadii=[1 1 1]  EllipsoidRadiiUnits=m  ExtrusionCrossSection=[1 1; -1 1; -1 -1; 1 -1]  ExtrusionCrossSectionUnits=m  ExtrusionLength=1  ExtrusionLengthUnits=m  PolygonNumSides=3  PolygonOuterRadius=1  PolygonOuterRadiusUnits=m  ExtGeomFileName=Hexagon_Socket_Button_Head_Screw_M3x6_Default_sldprt.STL  ExtGeomFileUnits=cm  RevolutionCrossSection=[1 1; 1 -1; 2 -1; 2 1]  RevolutionCrossSectionUnits=m  RevolutionExtent=Full  RevolutionAngle=180  RevolutionAngleUnits=deg  BlockFunction=simmechanics.library.body_elements.solid
  F : PMIOPort  Port=1  Side=Left
  connections:
  Solid/RConn1 -- ReferenceFrame/RConn1 -- F/RConn1

== system stewart_platform/ActuatorAssm5_2/CarrierAssm_1_RIGID/Hexagon_Socket_Button_Head_Screw_M3x6_3_RIGID ==
  ReferenceFrame : sm_lib/Frames and  Transforms/Reference  Frame  BlockFunction=simmechanics.library.frames_transforms.reference_frame
  Solid : sm_lib/Body Elements/Solid  InertiaType=Custom  Mass=0.00056348200000000002  MassUnits=kg  CenterOfMass=[0.143563 8.1476600000000005e-06 5.87883e-08]  CenterOfMassUnits=cm  MomentsOfInertia=[1.3098999999999999e-05 3.5078399999999999e-05 3.5077400000000004e-05]  MomentsOfInertiaUnits=kg*cm^2  ProductsOfInertia=[6.7519100000000001e-11 -7.6873799999999995e-12 -1.06542e-09]  ProductsOfInertiaUnits=kg*cm^2  DensityBased=on  Density=1000  DensityUnits=kg/(m^3)  GraphicType=FromGeometry  MarkerShape=Sphere  MarkerSize=10  MarkerSizeUnits=m  GraphicVisPropType=SimpleVisualProperties  GraphicDiffuseColor=[0.722824 0.722824 0.722824]  GraphicSpecularColor=[0.5 0.5 0.5 1.0]  GraphicAmbientColor=[0.15 0.15 0.15 1.0]  GraphicEmissiveColor=[0.0 0.0 0.0 1.0]  GraphicShininess=75  GraphicOpacity=1  GeometryShape=FromFile  RectangleSize=[1 1]  RectangleSizeUnits=m  BrickDimensions=[1 1 1]  BrickDimensionUnits=m  CylinderRadius=1  CylinderRadiusUnits=m  CylinderLength=1  CylinderLengthUnits=m  SphereRadius=1  SphereRadiusUnits=m  EllipsoidRadii=[1 1 1]  EllipsoidRadiiUnits=m  ExtrusionCrossSection=[1 1; -1 1; -1 -1; 1 -1]  ExtrusionCrossSectionUnits=m  ExtrusionLength=1  ExtrusionLengthUnits=m  PolygonNumSides=3  PolygonOuterRadius=1  PolygonOuterRadiusUnits=m  ExtGeomFileName=Hexagon_Socket_Button_Head_Screw_M3x6_Default_sldprt.STL  ExtGeomFileUnits=cm  RevolutionCrossSection=[1 1; 1 -1; 2 -1; 2 1]  RevolutionCrossSectionUnits=m  RevolutionExtent=Full  RevolutionAngle=180  RevolutionAngleUnits=deg  BlockFunction=simmechanics.library.body_elements.solid
  F : PMIOPort  Port=1  Side=Left
  connections:
  Solid/RConn1 -- ReferenceFrame/RConn1 -- F/RConn1

== system stewart_platform/ActuatorAssm5_2/CarrierAssm_1_RIGID/Hexagon_Socket_Button_Head_Screw_M3x6_4_RIGID ==
  ReferenceFrame : sm_lib/Frames and  Transforms/Reference  Frame  BlockFunction=simmechanics.library.frames_transforms.reference_frame
  Solid : sm_lib/Body Elements/Solid  InertiaType=Custom  Mass=0.00056348200000000002  MassUnits=kg  CenterOfMass=[0.143563 8.1476600000000005e-06 5.87883e-08]  CenterOfMassUnits=cm  MomentsOfInertia=[1.3098999999999999e-05 3.5078399999999999e-05 3.5077400000000004e-05]  MomentsOfInertiaUnits=kg*cm^2  ProductsOfInertia=[6.7519100000000001e-11 -7.6873799999999995e-12 -1.06542e-09]  ProductsOfInertiaUnits=kg*cm^2  DensityBased=on  Density=1000  DensityUnits=kg/(m^3)  GraphicType=FromGeometry  MarkerShape=Sphere  MarkerSize=10  MarkerSizeUnits=m  GraphicVisPropType=SimpleVisualProperties  GraphicDiffuseColor=[0.722824 0.722824 0.722824]  GraphicSpecularColor=[0.5 0.5 0.5 1.0]  GraphicAmbientColor=[0.15 0.15 0.15 1.0]  GraphicEmissiveColor=[0.0 0.0 0.0 1.0]  GraphicShininess=75  GraphicOpacity=1  GeometryShape=FromFile  RectangleSize=[1 1]  RectangleSizeUnits=m  BrickDimensions=[1 1 1]  BrickDimensionUnits=m  CylinderRadius=1  CylinderRadiusUnits=m  CylinderLength=1  CylinderLengthUnits=m  SphereRadius=1  SphereRadiusUnits=m  EllipsoidRadii=[1 1 1]  EllipsoidRadiiUnits=m  ExtrusionCrossSection=[1 1; -1 1; -1 -1; 1 -1]  ExtrusionCrossSectionUnits=m  ExtrusionLength=1  ExtrusionLengthUnits=m  PolygonNumSides=3  PolygonOuterRadius=1  PolygonOuterRadiusUnits=m  ExtGeomFileName=Hexagon_Socket_Button_Head_Screw_M3x6_Default_sldprt.STL  ExtGeomFileUnits=cm  RevolutionCrossSection=[1 1; 1 -1; 2 -1; 2 1]  RevolutionCrossSectionUnits=m  RevolutionExtent=Full  RevolutionAngle=180  RevolutionAngleUnits=deg  BlockFunction=simmechanics.library.body_elements.solid
  F : PMIOPort  Port=1  Side=Left
  connections:
  Solid/RConn1 -- ReferenceFrame/RConn1 -- F/RConn1

== system stewart_platform/ActuatorAssm5_2/CarrierAssm_1_RIGID/Hexagon_Socket_Button_Head_Screw_M3x6_5_RIGID ==
  ReferenceFrame : sm_lib/Frames and  Transforms/Reference  Frame  BlockFunction=simmechanics.library.frames_transforms.reference_frame
  Solid : sm_lib/Body Elements/Solid  InertiaType=Custom  Mass=0.00056348200000000002  MassUnits=kg  CenterOfMass=[0.143563 8.1476600000000005e-06 5.87883e-08]  CenterOfMassUnits=cm  MomentsOfInertia=[1.3098999999999999e-05 3.5078399999999999e-05 3.5077400000000004e-05]  MomentsOfInertiaUnits=kg*cm^2  ProductsOfInertia=[6.7519100000000001e-11 -7.6873799999999995e-12 -1.06542e-09]  ProductsOfInertiaUnits=kg*cm^2  DensityBased=on  Density=1000  DensityUnits=kg/(m^3)  GraphicType=FromGeometry  MarkerShape=Sphere  MarkerSize=10  MarkerSizeUnits=m  GraphicVisPropType=SimpleVisualProperties  GraphicDiffuseColor=[0.722824 0.722824 0.722824]  GraphicSpecularColor=[0.5 0.5 0.5 1.0]  GraphicAmbientColor=[0.15 0.15 0.15 1.0]  GraphicEmissiveColor=[0.0 0.0 0.0 1.0]  GraphicShininess=75  GraphicOpacity=1  GeometryShape=FromFile  RectangleSize=[1 1]  RectangleSizeUnits=m  BrickDimensions=[1 1 1]  BrickDimensionUnits=m  CylinderRadius=1  CylinderRadiusUnits=m  CylinderLength=1  CylinderLengthUnits=m  SphereRadius=1  SphereRadiusUnits=m  EllipsoidRadii=[1 1 1]  EllipsoidRadiiUnits=m  ExtrusionCrossSection=[1 1; -1 1; -1 -1; 1 -1]  ExtrusionCrossSectionUnits=m  ExtrusionLength=1  ExtrusionLengthUnits=m  PolygonNumSides=3  PolygonOuterRadius=1  PolygonOuterRadiusUnits=m  ExtGeomFileName=Hexagon_Socket_Button_Head_Screw_M3x6_Default_sldprt.STL  ExtGeomFileUnits=cm  RevolutionCrossSection=[1 1; 1 -1; 2 -1; 2 1]  RevolutionCrossSectionUnits=m  RevolutionExtent=Full  RevolutionAngle=180  RevolutionAngleUnits=deg  BlockFunction=simmechanics.library.body_elements.solid
  F : PMIOPort  Port=1  Side=Left
  connections:
  Solid/RConn1 -- ReferenceFrame/RConn1 -- F/RConn1

== system stewart_platform/ActuatorAssm5_2/CarrierAssm_1_RIGID/Hexagon_Socket_Button_Head_Screw_M3x6_6_RIGID ==
  ReferenceFrame : sm_lib/Frames and  Transforms/Reference  Frame  BlockFunction=simmechanics.library.frames_transforms.reference_frame
  Solid : sm_lib/Body Elements/Solid  InertiaType=Custom  Mass=0.00056348200000000002  MassUnits=kg  CenterOfMass=[0.143563 8.1476600000000005e-06 5.87883e-08]  CenterOfMassUnits=cm  MomentsOfInertia=[1.3098999999999999e-05 3.5078399999999999e-05 3.5077400000000004e-05]  MomentsOfInertiaUnits=kg*cm^2  ProductsOfInertia=[6.7519100000000001e-11 -7.6873799999999995e-12 -1.06542e-09]  ProductsOfInertiaUnits=kg*cm^2  DensityBased=on  Density=1000  DensityUnits=kg/(m^3)  GraphicType=FromGeometry  MarkerShape=Sphere  MarkerSize=10  MarkerSizeUnits=m  GraphicVisPropType=SimpleVisualProperties  GraphicDiffuseColor=[0.722824 0.722824 0.722824]  GraphicSpecularColor=[0.5 0.5 0.5 1.0]  GraphicAmbientColor=[0.15 0.15 0.15 1.0]  GraphicEmissiveColor=[0.0 0.0 0.0 1.0]  GraphicShininess=75  GraphicOpacity=1  GeometryShape=FromFile  RectangleSize=[1 1]  RectangleSizeUnits=m  BrickDimensions=[1 1 1]  BrickDimensionUnits=m  CylinderRadius=1  CylinderRadiusUnits=m  CylinderLength=1  CylinderLengthUnits=m  SphereRadius=1  SphereRadiusUnits=m  EllipsoidRadii=[1 1 1]  EllipsoidRadiiUnits=m  ExtrusionCrossSection=[1 1; -1 1; -1 -1; 1 -1]  ExtrusionCrossSectionUnits=m  ExtrusionLength=1  ExtrusionLengthUnits=m  PolygonNumSides=3  PolygonOuterRadius=1  PolygonOuterRadiusUnits=m  ExtGeomFileName=Hexagon_Socket_Button_Head_Screw_M3x6_Default_sldprt.STL  ExtGeomFileUnits=cm  RevolutionCrossSection=[1 1; 1 -1; 2 -1; 2 1]  RevolutionCrossSectionUnits=m  RevolutionExtent=Full  RevolutionAngle=180  RevolutionAngleUnits=deg  BlockFunction=simmechanics.library.body_elements.solid
  F : PMIOPort  Port=1  Side=Left
  connections:
  Solid/RConn1 -- ReferenceFrame/RConn1 -- F/RConn1

== system stewart_platform/ActuatorAssm5_2/CarrierAssm_1_RIGID/Hexagon_Socket_Button_Head_Screw_M3x6_7_RIGID ==
  ReferenceFrame : sm_lib/Frames and  Transforms/Reference  Frame  BlockFunction=simmechanics.library.frames_transforms.reference_frame
  Solid : sm_lib/Body Elements/Solid  InertiaType=Custom  Mass=0.00056348200000000002  MassUnits=kg  CenterOfMass=[0.143563 8.1476600000000005e-06 5.87883e-08]  CenterOfMassUnits=cm  MomentsOfInertia=[1.3098999999999999e-05 3.5078399999999999e-05 3.5077400000000004e-05]  MomentsOfInertiaUnits=kg*cm^2  ProductsOfInertia=[6.7519100000000001e-11 -7.6873799999999995e-12 -1.06542e-09]  ProductsOfInertiaUnits=kg*cm^2  DensityBased=on  Density=1000  DensityUnits=kg/(m^3)  GraphicType=FromGeometry  MarkerShape=Sphere  MarkerSize=10  MarkerSizeUnits=m  GraphicVisPropType=SimpleVisualProperties  GraphicDiffuseColor=[0.722824 0.722824 0.722824]  GraphicSpecularColor=[0.5 0.5 0.5 1.0]  GraphicAmbientColor=[0.15 0.15 0.15 1.0]  GraphicEmissiveColor=[0.0 0.0 0.0 1.0]  GraphicShininess=75  GraphicOpacity=1  GeometryShape=FromFile  RectangleSize=[1 1]  RectangleSizeUnits=m  BrickDimensions=[1 1 1]  BrickDimensionUnits=m  CylinderRadius=1  CylinderRadiusUnits=m  CylinderLength=1  CylinderLengthUnits=m  SphereRadius=1  SphereRadiusUnits=m  EllipsoidRadii=[1 1 1]  EllipsoidRadiiUnits=m  ExtrusionCrossSection=[1 1; -1 1; -1 -1; 1 -1]  ExtrusionCrossSectionUnits=m  ExtrusionLength=1  ExtrusionLengthUnits=m  PolygonNumSides=3  PolygonOuterRadius=1  PolygonOuterRadiusUnits=m  ExtGeomFileName=Hexagon_Socket_Button_Head_Screw_M3x6_Default_sldprt.STL  ExtGeomFileUnits=cm  RevolutionCrossSection=[1 1; 1 -1; 2 -1; 2 1]  RevolutionCrossSectionUnits=m  RevolutionExtent=Full  RevolutionAngle=180  RevolutionAngleUnits=deg  BlockFunction=simmechanics.library.body_elements.solid
  F : PMIOPort  Port=1  Side=Left
  connections:
  Solid/RConn1 -- ReferenceFrame/RConn1 -- F/RConn1

== system stewart_platform/ActuatorAssm5_2/CarrierAssm_1_RIGID/Hexagon_Socket_Button_Head_Screw_M3x6_8_RIGID ==
  ReferenceFrame : sm_lib/Frames and  Transforms/Reference  Frame  BlockFunction=simmechanics.library.frames_transforms.reference_frame
  Solid : sm_lib/Body Elements/Solid  InertiaType=Custom  Mass=0.00056348200000000002  MassUnits=kg  CenterOfMass=[0.143563 8.1476600000000005e-06 5.87883e-08]  CenterOfMassUnits=cm  MomentsOfInertia=[1.3098999999999999e-05 3.5078399999999999e-05 3.5077400000000004e-05]  MomentsOfInertiaUnits=kg*cm^2  ProductsOfInertia=[6.7519100000000001e-11 -7.6873799999999995e-12 -1.06542e-09]  ProductsOfInertiaUnits=kg*cm^2  DensityBased=on  Density=1000  DensityUnits=kg/(m^3)  GraphicType=FromGeometry  MarkerShape=Sphere  MarkerSize=10  MarkerSizeUnits=m  GraphicVisPropType=SimpleVisualProperties  GraphicDiffuseColor=[0.722824 0.722824 0.722824]  GraphicSpecularColor=[0.5 0.5 0.5 1.0]  GraphicAmbientColor=[0.15 0.15 0.15 1.0]  GraphicEmissiveColor=[0.0 0.0 0.0 1.0]  GraphicShininess=75  GraphicOpacity=1  GeometryShape=FromFile  RectangleSize=[1 1]  RectangleSizeUnits=m  BrickDimensions=[1 1 1]  BrickDimensionUnits=m  CylinderRadius=1  CylinderRadiusUnits=m  CylinderLength=1  CylinderLengthUnits=m  SphereRadius=1  SphereRadiusUnits=m  EllipsoidRadii=[1 1 1]  EllipsoidRadiiUnits=m  ExtrusionCrossSection=[1 1; -1 1; -1 -1; 1 -1]  ExtrusionCrossSectionUnits=m  ExtrusionLength=1  ExtrusionLengthUnits=m  PolygonNumSides=3  PolygonOuterRadius=1  PolygonOuterRadiusUnits=m  ExtGeomFileName=Hexagon_Socket_Button_Head_Screw_M3x6_Default_sldprt.STL  ExtGeomFileUnits=cm  RevolutionCrossSection=[1 1; 1 -1; 2 -1; 2 1]  RevolutionCrossSectionUnits=m  RevolutionExtent=Full  RevolutionAngle=180  RevolutionAngleUnits=deg  BlockFunction=simmechanics.library.body_elements.solid
  F : PMIOPort  Port=1  Side=Left
  connections:
  Solid/RConn1 -- ReferenceFrame/RConn1 -- F/RConn1

== system stewart_platform/ActuatorAssm5_2/CarrierAssm_1_RIGID/Hexagon_Socket_Head_Cap_Screw_M3x5_1_RIGID ==
  ReferenceFrame : sm_lib/Frames and  Transforms/Reference  Frame  BlockFunction=simmechanics.library.frames_transforms.reference_frame
  Solid : sm_lib/Body Elements/Solid  InertiaType=Custom  Mass=0.00075563799999999999  MassUnits=kg  CenterOfMass=[-0.00070356100000000001 3.3976700000000003e-05 2.42889e-07]  CenterOfMassUnits=cm  MomentsOfInertia=[2.3283100000000001e-05 4.6861000000000004e-05 4.6851300000000003e-05]  MomentsOfInertiaUnits=kg*cm^2  ProductsOfInertia=[6.6364300000000002e-10 -4.0249100000000001e-11 -5.63026e-09]  ProductsOfInertiaUnits=kg*cm^2  DensityBased=on  Density=1000  DensityUnits=kg/(m^3)  GraphicType=FromGeometry  MarkerShape=Sphere  MarkerSize=10  MarkerSizeUnits=m  GraphicVisPropType=SimpleVisualProperties  GraphicDiffuseColor=[0.722824 0.722824 0.722824]  GraphicSpecularColor=[0.5 0.5 0.5 1.0]  GraphicAmbientColor=[0.15 0.15 0.15 1.0]  GraphicEmissiveColor=[0.0 0.0 0.0 1.0]  GraphicShininess=75  GraphicOpacity=1  GeometryShape=FromFile  RectangleSize=[1 1]  RectangleSizeUnits=m  BrickDimensions=[1 1 1]  BrickDimensionUnits=m  CylinderRadius=1  CylinderRadiusUnits=m  CylinderLength=1  CylinderLengthUnits=m  SphereRadius=1  SphereRadiusUnits=m  EllipsoidRadii=[1 1 1]  EllipsoidRadiiUnits=m  ExtrusionCrossSection=[1 1; -1 1; -1 -1; 1 -1]  ExtrusionCrossSectionUnits=m  ExtrusionLength=1  ExtrusionLengthUnits=m  PolygonNumSides=3  PolygonOuterRadius=1  PolygonOuterRadiusUnits=m  ExtGeomFileName=Hexagon_Socket_Head_Cap_Screw_M3x5_Default_sldprt.STL  ExtGeomFileUnits=cm  RevolutionCrossSection=[1 1; 1 -1; 2 -1; 2 1]  RevolutionCrossSectionUnits=m  RevolutionExtent=Full  RevolutionAngle=180  RevolutionAngleUnits=deg  BlockFunction=simmechanics.library.body_elements.solid
  F : PMIOPort  Port=1  Side=Left
  connections:
  Solid/RConn1 -- ReferenceFrame/RConn1 -- F/RConn1

== system stewart_platform/ActuatorAssm5_2/CarrierAssm_1_RIGID/Hexagon_Socket_Head_Cap_Screw_M3x5_2_RIGID ==
  ReferenceFrame : sm_lib/Frames and  Transforms/Reference  Frame  BlockFunction=simmechanics.library.frames_transforms.reference_frame
  Solid : sm_lib/Body Elements/Solid  InertiaType=Custom  Mass=0.00075563799999999999  MassUnits=kg  CenterOfMass=[-0.00070356100000000001 3.3976700000000003e-05 2.42889e-07]  CenterOfMassUnits=cm  MomentsOfInertia=[2.3283100000000001e-05 4.6861000000000004e-05 4.6851300000000003e-05]  MomentsOfInertiaUnits=kg*cm^2  ProductsOfInertia=[6.6364300000000002e-10 -4.0249100000000001e-11 -5.63026e-09]  ProductsOfInertiaUnits=kg*cm^2  DensityBased=on  Density=1000  DensityUnits=kg/(m^3)  GraphicType=FromGeometry  MarkerShape=Sphere  MarkerSize=10  MarkerSizeUnits=m  GraphicVisPropType=SimpleVisualProperties  GraphicDiffuseColor=[0.722824 0.722824 0.722824]  GraphicSpecularColor=[0.5 0.5 0.5 1.0]  GraphicAmbientColor=[0.15 0.15 0.15 1.0]  GraphicEmissiveColor=[0.0 0.0 0.0 1.0]  GraphicShininess=75  GraphicOpacity=1  GeometryShape=FromFile  RectangleSize=[1 1]  RectangleSizeUnits=m  BrickDimensions=[1 1 1]  BrickDimensionUnits=m  CylinderRadius=1  CylinderRadiusUnits=m  CylinderLength=1  CylinderLengthUnits=m  SphereRadius=1  SphereRadiusUnits=m  EllipsoidRadii=[1 1 1]  EllipsoidRadiiUnits=m  ExtrusionCrossSection=[1 1; -1 1; -1 -1; 1 -1]  ExtrusionCrossSectionUnits=m  ExtrusionLength=1  ExtrusionLengthUnits=m  PolygonNumSides=3  PolygonOuterRadius=1  PolygonOuterRadiusUnits=m  ExtGeomFileName=Hexagon_Socket_Head_Cap_Screw_M3x5_Default_sldprt.STL  ExtGeomFileUnits=cm  RevolutionCrossSection=[1 1; 1 -1; 2 -1; 2 1]  RevolutionCrossSectionUnits=m  RevolutionExtent=Full  RevolutionAngle=180  RevolutionAngleUnits=deg  BlockFunction=simmechanics.library.body_elements.solid
  F : PMIOPort  Port=1  Side=Left
  connections:
  Solid/RConn1 -- ReferenceFrame/RConn1 -- F/RConn1
